simulink model "mqr_att"  (R2019a)
settings: Solver=VariableStepAuto  StartTime=0.0  StopTime=100  RelTol=1e-3
undefined symbols (not defined in the file): den, num
settings Model: Creator=tarci  LastModifiedBy=PICHAU
settings DataIOCC: ReturnWorkspaceOutputs=off
settings DebuggingCC: ArithmeticOperatorsInVariantConditions=warning

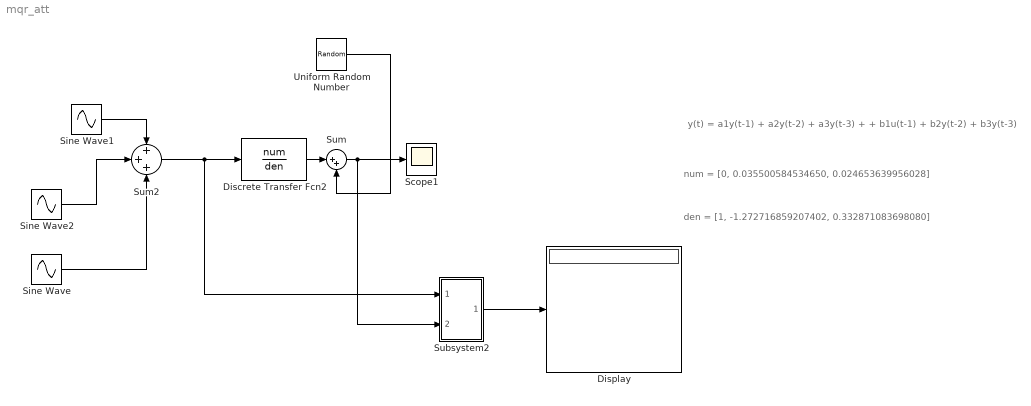
== system mqr_att ==
  note: y(t) = a1y(t-1) + a2y(t-2) + a3y(t-3) + + b1u(t-1) + b2y(t-2) + b3y(t-3)
  note: den = [1, -1.272716859207402, 0.332871083698080]
  note: num = [0, 0.035500584534650, 0.024653639956028]
  Discrete Transfer Fcn2 : DiscreteTransferFcn  Numerator=num  Denominator=den  SampleTime=0.1
  Display : Display
  Scope1 : Scope
  Sine Wave : Sin  SampleTime=0
  Sine Wave1 : Sin  Amplitude=2  Frequency=0.5  SampleTime=0
  Sine Wave2 : Sin  Frequency=0.1  SampleTime=0
  Subsystem2 : Subsystem
  Sum : Sum  Inputs=|++
  Sum2 : Sum  Inputs=+++
  Uniform Random Number : UniformRandomNumber  Minimum=-0.01  Maximum=0.01  SampleTime=0.1
  wires:
  Subsystem2/1(Out1) -> Display/1
  Discrete Transfer Fcn2/1 -> Sum/1
  Sum2/1 -> Subsystem2/1(In1), Discrete Transfer Fcn2/1
  Sum/1 -> Subsystem2/2(In2), Scope1/1
  Uniform Random Number/1 -> Sum/2
  Sine Wave1/1 -> Sum2/1
  Sine Wave2/1 -> Sum2/2
  Sine Wave/1 -> Sum2/3

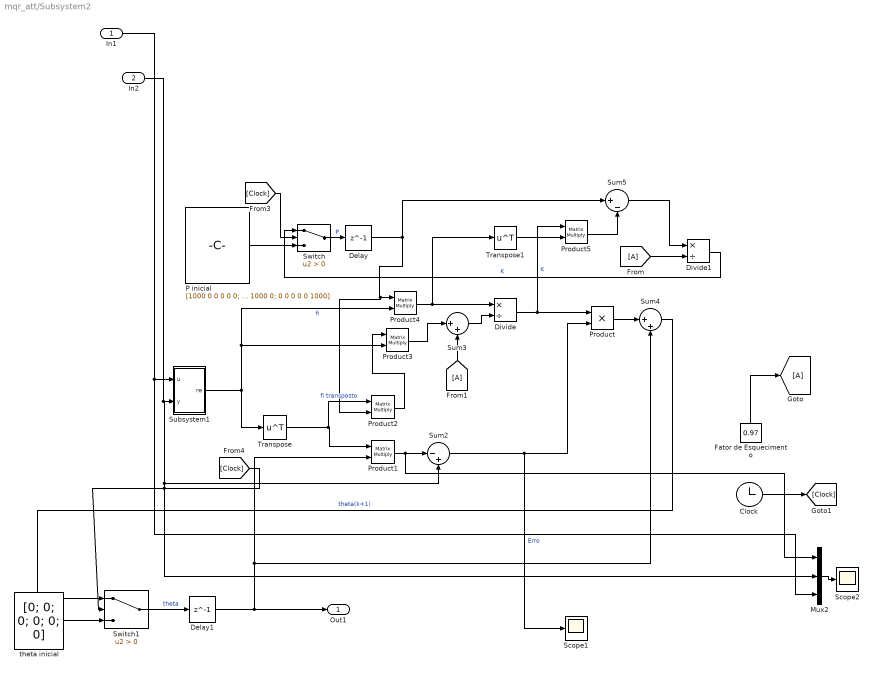
== system mqr_att/Subsystem2 ==
  In1 : Inport
  In2 : Inport  Port=2
  Clock : Clock
  Delay : Delay  DelayLength=1  InitialCondition=0  SampleTime=0.1
  Delay1 : Delay  DelayLength=1  InitialCondition=0  SampleTime=0.1
  Divide : Product  Inputs=*/
  Divide1 : Product  Inputs=*/
  "Fator de Esquecimento " : Constant  Value=0.97
  Mux2 : Mux  Inputs=3
  P inicial : Constant  Value=[1000 0 0 0 0 0; 0 1000 0 0 0 0; 0 0 1000 0 0 0; 0 0 0 1000 0 0; 0 0 0 0 1000 0; 0 0 0 0 0 1000]
  Product : Product
  Product{1..5} (5 alike) : Product  Multiplication=Matrix(*)
  Scope1 : Scope
  Scope2 : Scope
  Subsystem1 : Subsystem
  Sum2 : Sum  Inputs=|-+
  Sum3 : Sum  Inputs=|++
  Sum4 : Sum  Inputs=|++
  Sum5 : Sum  Inputs=|+-
  Switch : Switch  Criteria=u2 > Threshold
  Switch1 : Switch  Criteria=u2 > Threshold
  Transpose : Math  Operator=transpose  SaturateOnIntegerOverflow=on
  Transpose1 : Math  Operator=transpose  SaturateOnIntegerOverflow=on
  "theta inicial " : Constant  Value=[0; 0; 0; 0; 0; 0]
  Out1 : Outport
  wires:
  Subsystem1/1(re) -> Transpose/1, Product4/2, Product3/2  "fi"
  Product/1 -> Sum4/1
  In2/1 -> Mux2/2, Sum2/2, Subsystem1/2(y)
  "Fator de Esquecimento "/1 -> [A]
  Transpose/1 -> Product2/1, Product1/1  "fi transposto"
  Sum3/1 -> Divide/2
  Product3/1 -> Sum3/1
  Switch/1 -> Delay/1  "P"
  Product4/1 -> Transpose1/1, Divide/1
  Delay/1 -> Product2/2, Product4/1, Sum5/1
  Divide/1 -> Product5/1, Product/1  "K"
  Transpose1/1 -> Product5/2
  Sum5/1 -> Divide1/1
  Sum2/1 -> Scope1/1, Product/2  "Erro"
  Delay1/1 -> Sum4/2, Product1/2, Out1/1
  Divide1/1 -> Switch/1  "K"
  "theta inicial "/1 -> Switch1/3
  [A] -> Divide1/2
  Product2/1 -> Product3/1
  [Clock] -> Switch1/2
  Clock/1 -> [Clock]
  Product1/1 -> Mux2/1, Sum2/1
  Product5/1 -> Sum5/2
  P inicial/1 -> Switch/3
  Sum4/1 -> Switch1/1  "theta(k+1)"
  [A] -> Sum3/2
  In1/1 -> Mux2/3, Subsystem1/1(u)
  [Clock] -> Switch/2
  Switch1/1 -> Delay1/1  "theta"
  Mux2/1 -> Scope2/1

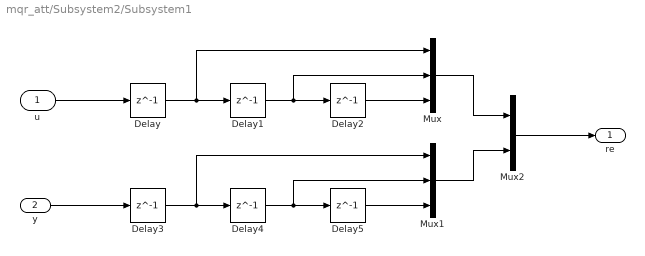
== system mqr_att/Subsystem2/Subsystem1 ==
  u : Inport
  y : Inport  Port=2
  Delay{,1..5} (6 alike) : Delay  DelayLength=1  InitialCondition=0  SampleTime=0.1
  Mux : Mux  Inputs=3
  Mux1 : Mux  Inputs=3
  Mux2 : Mux  Inputs=2
  re : Outport
  wires:
  Delay4/1 -> Mux1/2, Delay5/1
  u/1 -> Delay/1
  Delay5/1 -> Mux1/3
  Delay/1 -> Mux/1, Delay1/1
  Mux1/1 -> Mux2/2
  Delay1/1 -> Mux/2, Delay2/1
  Mux/1 -> Mux2/1
  Mux2/1 -> re/1
  Delay3/1 -> Mux1/1, Delay4/1
  Delay2/1 -> Mux/3
  y/1 -> Delay3/1
